simulink model "code_group35"  (R2020a)
settings: Solver=FixedStepAuto  StartTime=0.0  StopTime=10.0  FixedStep=1e-3  RelTol=1e-3  EnableMultiTasking=on
undefined symbols (not defined in the file): A0, A1, D0, D1, D10, D11, D12, D13, D2, D3, D4, D5, D6, D7, D8, D9, PTA0, PTA1, PTA2, PTB2, PTB23, PTB3, PTB9, PTC16, PTC17, PTC2, PTC3, PTC4, PTD0, PTD1, PTD2, PTD3
libraries: frdmk64flib x25, etargetslib x6, dspstat3 x1
settings Model: ExtModeTrigDuration=5  Creator=braed  LastModifiedBy=braed
settings OptimizationCC: EnhancedBackFolding=on  PassReuseOutputArgsAs=Individual arguments  ZeroExternalMemoryAtStartup=off  ZeroInternalMemoryAtStartup=off  MaxStackSize=64  OptimizeBlockOrder=speed  DifferentSizesBufferReuse=on  OptimizationCustomize=off  EfficientTunableParamExpr=on
settings DebuggingCC: ParameterTunabilityLossMsg=error
settings HardwareCC: ProdBitPerPointer=32  ProdBitPerSizeT=32  ProdBitPerPtrDiffT=32  ProdLargestAtomicInteger=Long  ProdLargestAtomicFloat=Double  ProdWordSize=32  ProdHWDeviceType=ARM Compatible->ARM Cortex
settings SFSimCC: MATLABDynamicMemAlloc=off
settings RTWCC: SystemTargetFile=ert.tlc  HardwareBoard=NXP FRDM-K64F  TemplateMakefile=ert_default_tmf  Toolchain=GNU Tools for ARM Embedded Processors
settings CodeAppCC: ForceParamTrailComments=on  IgnoreCustomStorageClasses=off  OperatorAnnotations=on  SimulinkDataObjDesc=on  SFDataObjDesc=on  InsertBlockDesc=on

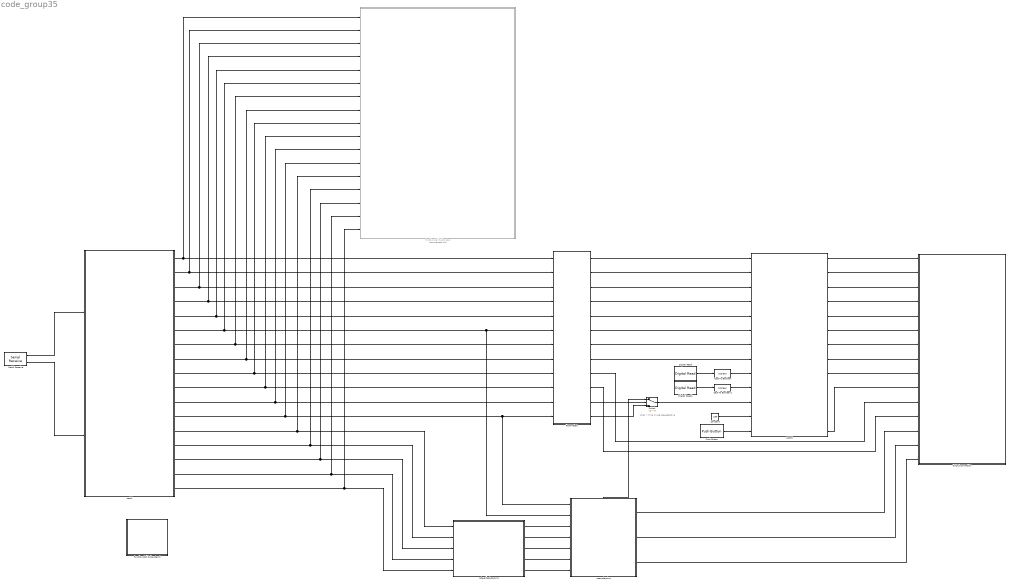
== system code_group35 ==
  note: when > 0 (ie 1) use rate_adaptive
  " Output connection" : Subsystem
  Cast To Boolean : DataTypeConversion  OutDataTypeStr=boolean
  Cast To Boolean1 : DataTypeConversion  OutDataTypeStr=boolean
  Constant : Constant  Value=250
  Digital Read : frdmk64flib/Digital Read  Whichpin=PTC16 (D0)  SampleTime=-1
  Digital Read1 : frdmk64flib/Digital Read  Whichpin=PTC17 (D1)  SampleTime=-1
  Function-Call Subsystem : Subsystem  Commented=on  TreatAsAtomicUnit=on
  Function-Call Subsystem1 : Subsystem  TreatAsAtomicUnit=on
  LOGIC : Stateflow chart  TreatAsAtomicUnit=on
  Parameters : Subsystem
  Push Button : frdmk64flib/Push Button  Whichswitch=SW2  SampleTime1=-1
  Serial Receive : frdmk64flib/Serial Receive  SCIModule=0  Baudrate=uint32(9600)  Parity=None  StopBits=1  HardwareFlowControl=None  ByteOrder=LittleEndian  DataType=uint8  DataLength=28  BlockingMode=off  OutputStatus=on  SampleTime=-1
  Switch : Switch  Criteria=u2 > Threshold
  rate adaptive : Subsystem
      settings: PortSchema="{\"entries\":[{\"content\":{\"sides\":[{\"content\":{\"connectorIds\":[\"In1\",\"In2\",\"In3\",\"In4\",\"In5\",\"In6\",\"In7\"]},\"type\":\"ConnectorPlacement.EquallySpacedRectSide\",\"uuid\":\"63ecb548-1bfe-492b-8fa1-384c5f75ccdd\"},{\"content\":{\"connectorIds\":[\"Out1\",\"Out2\",\"Out3\"],\"side\":\"RIGHT\"},\"type\":\"ConnectorPlacement.EquallySpacedRectSide\",\"uuid\":\"03d354e8-60bf-4739-8c68-3b2530a8d39d\"},{\"content\":{\"connectorIds\":[\"Out4\"],\"side\":\"TOP\"},\"type\":\"ConnectorPlacement.EquallySpacedRectSide\",\"uuid\":\"87bdc17e-9d8d-401e-9bc9-5c1e683b110d\"}]},\"type\":\"ConnectorPlacement.EquallySpacedConnector\",\"uuid\":\"8522751d-691b-4abf-a216-245af807604c\"}],\"packageUris\":[\"http://schema.mathworks.com/mf0/Connector/19700101\"],\"version\":\"1.0\"}"
  rate_adapt_params : Subsystem
  serial : Stateflow chart  TreatAsAtomicUnit=on
  wires:
  LOGIC/7(ATR_GND_CTRL) -> " Output connection"/7(ATR_GND_CTRL)
  Parameters/1(mode_out) -> LOGIC/1(mode)
  Parameters/6(upperInterval) -> LOGIC/6(upper_interval_rate)
  Parameters/7(ARP) -> LOGIC/7(ARP)
  Parameters/8(VRP) -> LOGIC/8(VRP)
  Parameters/5(vent_pulse_amp) -> LOGIC/5(vent_amp)
  Parameters/10(VentSensitivity) -> " Output connection"/12(VENT_CMP_REF_PWM)
  Parameters/2(atr_pulse_width) -> LOGIC/2(atr_pulse_width)
  Parameters/4(vent_pulse_width) -> LOGIC/4(vent_pulse_width)
  Parameters/9(AtrSensitivity) -> " Output connection"/11(ATR_CMP_REF_PWM)
  LOGIC/5(VENT_PACE_CTRL) -> " Output connection"/5(VENT_PACE_CTRL)
  Digital Read/1 -> Cast To Boolean/1
  Digital Read1/1 -> Cast To Boolean1/1
  Parameters/3(atr_pulse_amp) -> LOGIC/3(atr_amp)
  LOGIC/13(FRONTEND_CTRL) -> " Output connection"/10(FRONTEND_CTRL)
  Cast To Boolean/1 -> LOGIC/9(ATR_CMP_DETECT)
  Cast To Boolean1/1 -> LOGIC/10(VENT_CMP_DETECT)
  LOGIC/3(Z_VENT_CTRL) -> " Output connection"/3(Z_VENT_CTRL)
  LOGIC/4(ATR_PACE_CTRL) -> " Output connection"/4(ATR_PACE_CTRL)
  LOGIC/8(VENT_GND_CTRL) -> " Output connection"/8(VENT_GND_CTRL)
  LOGIC/9(PACE_CHARGE_CTRL) -> " Output connection"/9(PACE_CHARGE_CTRL)
  LOGIC/1(PACING_REF_PWM) -> " Output connection"/1(PACING_REF_PWM)
  LOGIC/2(Z_ATR_CTRL) -> " Output connection"/2(Z_ATR_CTRL)
  LOGIC/6(PACE_GND_CTRL) -> " Output connection"/6(PACE_GND_CTRL)
  Serial Receive/1 -> serial/1(rxdata)
  Serial Receive/2 -> serial/2(status)
  rate adaptive/3(led_b) -> " Output connection"/15(B_LED)
  rate adaptive/1(led_r) -> " Output connection"/13(R_LED)
  rate adaptive/2(led_g) -> " Output connection"/14(G_LED)
  Parameters/11(rate_adaptive_out) -> Switch/2
  rate adaptive/4(pacing_rate) -> Switch/1
  Parameters/12(lowerInterval) -> Switch/3
  Switch/1 -> LOGIC/11(lower_interval_rate)
  serial/1(mode) -> Function-Call Subsystem/1(mode), Parameters/1(mode_in)
  serial/2(atr_pw) -> Function-Call Subsystem/2(atr_pw), Parameters/2(atr_pw)
  serial/4(vent_pw) -> Function-Call Subsystem/4(vent_pw), Parameters/4(vent_pw)
  serial/5(vent_amp) -> Function-Call Subsystem/5(vent_amp), Parameters/5(vent_amp)
  serial/6(LRL) -> Function-Call Subsystem/6(LRL), rate adaptive/2(LRL_in), Parameters/6(lowerRateIn)
  serial/7(URL) -> Function-Call Subsystem/7(URL), Parameters/7(upperRateIn)
  serial/8(ARP) -> Function-Call Subsystem/8(ARP), Parameters/8(ARPIn)
  serial/9(VRP) -> Function-Call Subsystem/9(VRP), Parameters/9(VRPIn)
  serial/10(atr_sense) -> Function-Call Subsystem/10(atr_sense), Parameters/10(AtrSensitivityIn)
  serial/11(vent_sense) -> Function-Call Subsystem/11(vent_sense), Parameters/11(VentSensitivityIn)
  serial/12(rate_adp) -> Function-Call Subsystem/12(rate_adp), rate adaptive/1(rate_adaptive_in), Parameters/12(rate_adaptive_in)
  rate_adapt_params/1(MSRout) -> rate adaptive/3(MSR_in)
  rate_adapt_params/2(reac_out) -> rate adaptive/4(reac_time)
  rate_adapt_params/3(recov_out) -> rate adaptive/5(recov_time)
  rate_adapt_params/4(act_thresh_out) -> rate adaptive/6(activity_threshold)
  rate_adapt_params/5(resp_out) -> rate adaptive/7(response_factor)
  serial/13(MSR) -> Function-Call Subsystem/13(MSR), rate_adapt_params/1(MSRin)
  serial/15(recov_t) -> Function-Call Subsystem/15(recov_t), rate_adapt_params/3(recov_in)
  serial/16(act_thresh) -> Function-Call Subsystem/16(act_thresh), rate_adapt_params/4(act_thresh_in)
  serial/17(res_fact) -> Function-Call Subsystem/17(res_fact), rate_adapt_params/5(resp_in)
  serial/3(atr_amp) -> Function-Call Subsystem/3(atr_amp), Parameters/3(atr_amp)
  serial/14(reac_t) -> Function-Call Subsystem/14(reac_t), rate_adapt_params/2(reac_in)
  Constant/1 -> LOGIC/12(AV_Delay)
  Push Button/1 -> LOGIC/13(button)

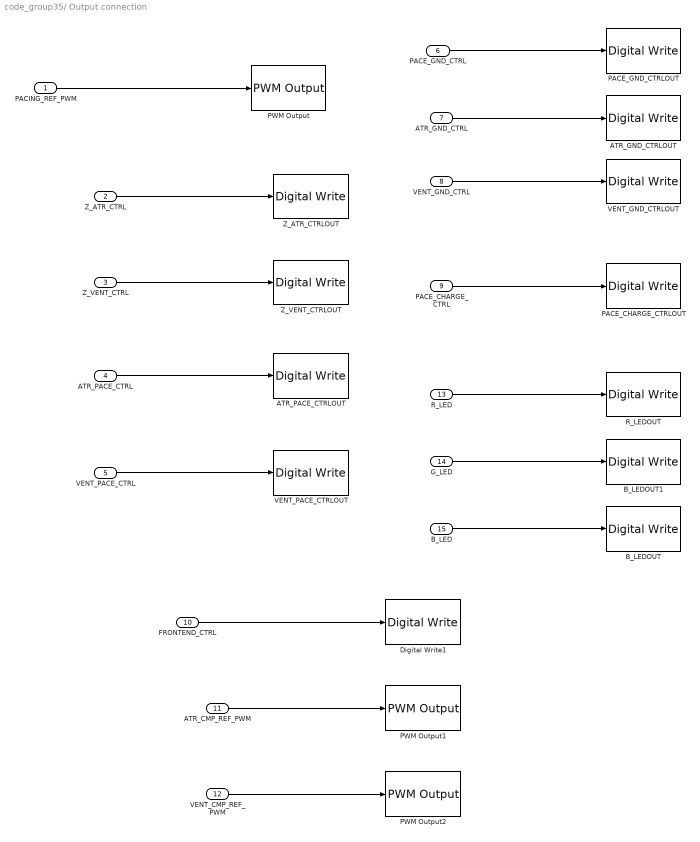
== system code_group35/ Output connection ==
  PACING_REF_PWM : Inport  OutDataTypeStr=uint32
  Z_ATR_CTRL : Inport  Port=2  OutDataTypeStr=uint32
  Z_VENT_CTRL : Inport  Port=3  OutDataTypeStr=uint32
  ATR_PACE_CTRL : Inport  Port=4  OutDataTypeStr=uint32
  VENT_PACE_CTRL : Inport  Port=5  OutDataTypeStr=uint32
  PACE_GND_CTRL : Inport  Port=6  OutDataTypeStr=uint32
  ATR_GND_CTRL : Inport  Port=7  OutDataTypeStr=uint32
  VENT_GND_CTRL : Inport  Port=8  OutDataTypeStr=uint32
  PACE_CHARGE_CTRL : Inport  Port=9  OutDataTypeStr=uint32
  FRONTEND_CTRL : Inport  Port=10  OutDataTypeStr=uint8
  ATR_CMP_REF_PWM : Inport  Port=11  OutDataTypeStr=uint32
  VENT_CMP_REF_PWM : Inport  Port=12  OutDataTypeStr=uint32
  R_LED : Inport  Port=13  OutDataTypeStr=uint32
  G_LED : Inport  Port=14  OutDataTypeStr=uint32
  B_LED : Inport  Port=15  OutDataTypeStr=uint32
  ATR_GND_CTRLOUT : frdmk64flib/Digital Write  Whichpin=PTD2 (D11)
  ATR_PACE_CTRLOUT : frdmk64flib/Digital Write  Whichpin=PTA0 (D8)
  B_LEDOUT : frdmk64flib/Digital Write  Whichpin=BLUE_LED
  B_LEDOUT1 : frdmk64flib/Digital Write  Whichpin=GREEN_LED
  Digital Write1 : frdmk64flib/Digital Write  Whichpin=PTD1 (D13)
  PACE_CHARGE_CTRLOUT : frdmk64flib/Digital Write  Whichpin=PTB9 (D2)
  PACE_GND_CTRLOUT : frdmk64flib/Digital Write  Whichpin=PTD0 (D10)
  PWM Output : frdmk64flib/PWM Output  Whichpin=PTA2 (D5)  InitialFrequency=2000  InitialDutyCycle=30
  PWM Output1 : frdmk64flib/PWM Output  Whichpin=PTC2 (D6)  InitialFrequency=2000  InitialDutyCycle=30
  PWM Output2 : frdmk64flib/PWM Output  Whichpin=PTA1 (D3)  InitialFrequency=2000  InitialDutyCycle=30
  R_LEDOUT : frdmk64flib/Digital Write  Whichpin=RED_LED
  VENT_GND_CTRLOUT : frdmk64flib/Digital Write  Whichpin=PTD3 (D12)
  VENT_PACE_CTRLOUT : frdmk64flib/Digital Write  Whichpin=PTC4 (D9)
  Z_ATR_CTRLOUT : frdmk64flib/Digital Write  Whichpin=PTB23 (D4)
  Z_VENT_CTRLOUT : frdmk64flib/Digital Write  Whichpin=PTC3 (D7)
  wires:
  PACING_REF_PWM/1 -> PWM Output/1
  Z_VENT_CTRL/1 -> Z_VENT_CTRLOUT/1
  PACE_GND_CTRL/1 -> PACE_GND_CTRLOUT/1
  Z_ATR_CTRL/1 -> Z_ATR_CTRLOUT/1
  ATR_PACE_CTRL/1 -> ATR_PACE_CTRLOUT/1
  VENT_GND_CTRL/1 -> VENT_GND_CTRLOUT/1
  B_LED/1 -> B_LEDOUT/1
  PACE_CHARGE_CTRL/1 -> PACE_CHARGE_CTRLOUT/1
  ATR_GND_CTRL/1 -> ATR_GND_CTRLOUT/1
  G_LED/1 -> B_LEDOUT1/1
  R_LED/1 -> R_LEDOUT/1
  VENT_PACE_CTRL/1 -> VENT_PACE_CTRLOUT/1
  VENT_CMP_REF_PWM/1 -> PWM Output2/1
  ATR_CMP_REF_PWM/1 -> PWM Output1/1
  FRONTEND_CTRL/1 -> Digital Write1/1

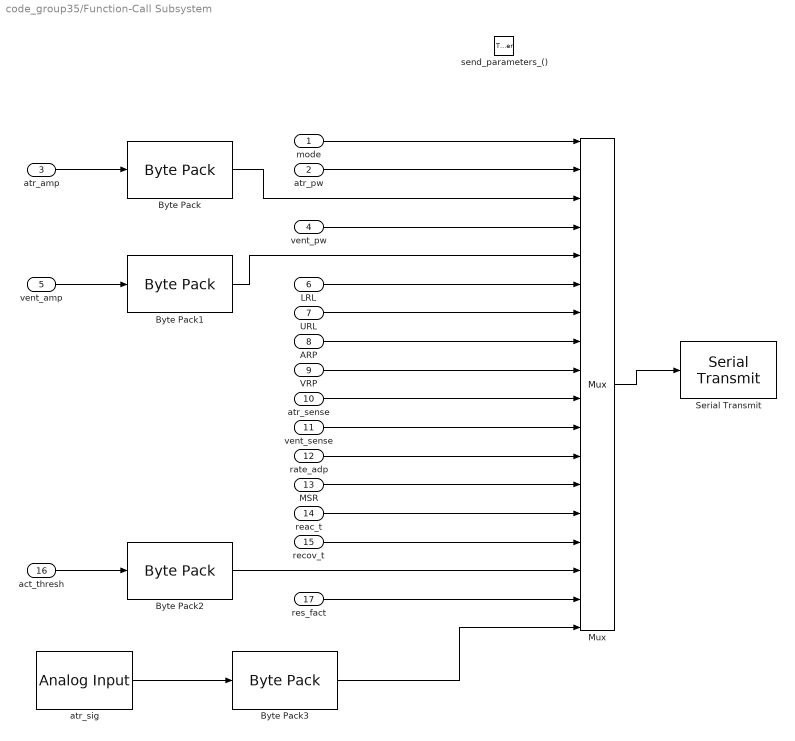
== system code_group35/Function-Call Subsystem ==
  mode : Inport
  atr_pw : Inport  Port=2
  atr_amp : Inport  Port=3
  vent_pw : Inport  Port=4
  vent_amp : Inport  Port=5
  LRL : Inport  Port=6
  URL : Inport  Port=7
  ARP : Inport  Port=8
  VRP : Inport  Port=9
  atr_sense : Inport  Port=10
  vent_sense : Inport  Port=11
  rate_adp : Inport  Port=12
  MSR : Inport  Port=13
  reac_t : Inport  Port=14
  recov_t : Inport  Port=15
  act_thresh : Inport  Port=16
  res_fact : Inport  Port=17
  send_parameters_() : TriggerPort  TriggerType=function-call  IsSimulinkFunction=on  FunctionName=send_parameters_  VariantControl=Variant
  Byte Pack : etargetslib/Byte Pack  datatypes={'single'}  byteAlign=1
  Byte Pack1 : etargetslib/Byte Pack  datatypes={'single'}  byteAlign=1
  Byte Pack2 : etargetslib/Byte Pack  datatypes={'single'}  byteAlign=1
  Byte Pack3 : etargetslib/Byte Pack  datatypes={'double'}  byteAlign=1
  Mux : Mux  Inputs=18
  Serial Transmit : frdmk64flib/Serial Transmit  SCIModule=0  Baudrate=uint32(9600)  Parity=None  StopBits=1  HardwareFlowControl=None  ByteOrder=LittleEndian  BlockingMode=on  OutputStatus=off
  atr_sig : frdmk64flib/Analog Input  Whichpin=PTB2 (A0)  SampleTime=-1
  wires:
  mode/1 -> Mux/1
  Mux/1 -> Serial Transmit/1
  atr_pw/1 -> Mux/2
  atr_amp/1 -> Byte Pack/1
  Byte Pack/1 -> Mux/3
  vent_pw/1 -> Mux/4
  LRL/1 -> Mux/6
  URL/1 -> Mux/7
  ARP/1 -> Mux/8
  VRP/1 -> Mux/9
  atr_sense/1 -> Mux/10
  vent_sense/1 -> Mux/11
  rate_adp/1 -> Mux/12
  MSR/1 -> Mux/13
  reac_t/1 -> Mux/14
  recov_t/1 -> Mux/15
  act_thresh/1 -> Byte Pack2/1
  res_fact/1 -> Mux/17
  Byte Pack1/1 -> Mux/5
  vent_amp/1 -> Byte Pack1/1
  Byte Pack2/1 -> Mux/16
  atr_sig/1 -> Byte Pack3/1
  Byte Pack3/1 -> Mux/18

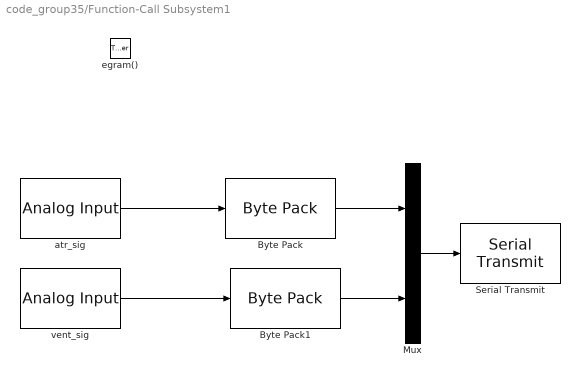
== system code_group35/Function-Call Subsystem1 ==
  egram() : TriggerPort  TriggerType=function-call  IsSimulinkFunction=on  FunctionName=egram_double  VariantControl=Variant
  Byte Pack : etargetslib/Byte Pack  datatypes={'double'}  byteAlign=1
  Byte Pack1 : etargetslib/Byte Pack  datatypes={'double'}  byteAlign=1
  Mux : Mux  Inputs=2
  Serial Transmit : frdmk64flib/Serial Transmit  SCIModule=0  Baudrate=uint32(9600)  Parity=None  StopBits=1  HardwareFlowControl=None  ByteOrder=LittleEndian  BlockingMode=on  OutputStatus=off
  atr_sig : frdmk64flib/Analog Input  Whichpin=PTB2 (A0)  SampleTime=-1
  vent_sig : frdmk64flib/Analog Input  Whichpin=PTB3 (A1)  SampleTime=-1
  wires:
  Mux/1 -> Serial Transmit/1
  atr_sig/1 -> Byte Pack/1
  vent_sig/1 -> Byte Pack1/1
  Byte Pack1/1 -> Mux/2
  Byte Pack/1 -> Mux/1

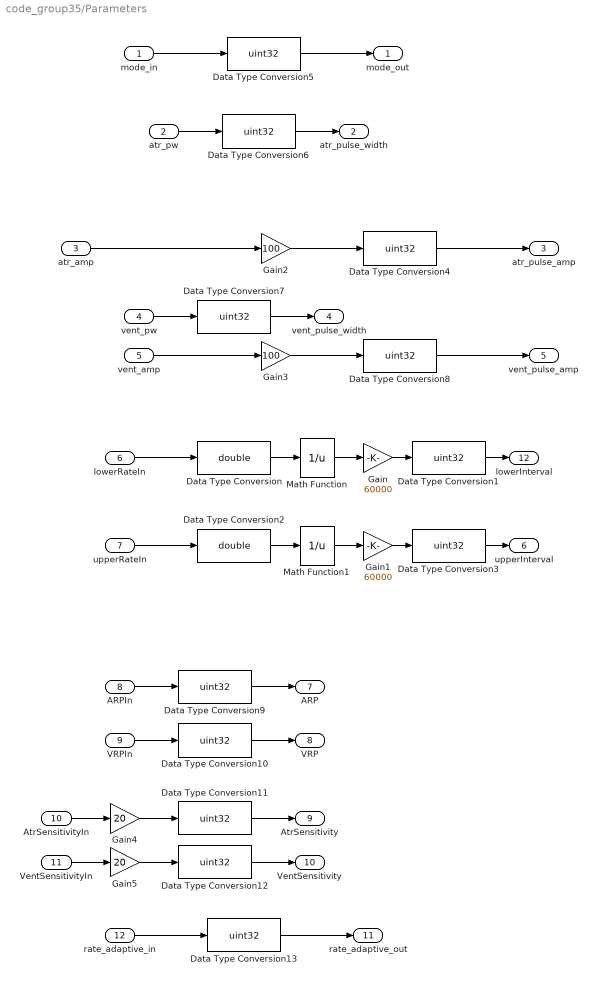
== system code_group35/Parameters ==
  mode_in : Inport  OutDataTypeStr=uint8
  atr_pw : Inport  Port=2  OutDataTypeStr=uint8
  atr_amp : Inport  Port=3  OutDataTypeStr=single
  vent_pw : Inport  Port=4  OutDataTypeStr=uint8
  vent_amp : Inport  Port=5  OutDataTypeStr=single
  lowerRateIn : Inport  Port=6  OutDataTypeStr=uint8  Unit=ppm
  upperRateIn : Inport  Port=7  OutDataTypeStr=uint8  Unit=ppm
  ARPIn : Inport  Port=8  OutDataTypeStr=uint8
  VRPIn : Inport  Port=9  OutDataTypeStr=uint8
  AtrSensitivityIn : Inport  Port=10  OutDataTypeStr=uint8
  VentSensitivityIn : Inport  Port=11  OutDataTypeStr=uint8
  rate_adaptive_in : Inport  Port=12  OutDataTypeStr=uint8
  Data Type Conversion : DataTypeConversion  OutDataTypeStr=double
  Data Type Conversion1 : DataTypeConversion  OutDataTypeStr=uint32
  Data Type Conversion{4..13} (10 alike) : DataTypeConversion  OutDataTypeStr=uint32  RndMeth=Round
  Data Type Conversion2 : DataTypeConversion  OutDataTypeStr=double
  Data Type Conversion3 : DataTypeConversion  OutDataTypeStr=uint32
  Gain : Gain  Gain=60000  OutDataTypeStr=double
  Gain1 : Gain  Gain=60000  OutDataTypeStr=double
  Gain2 : Gain  Gain=100  OutDataTypeStr=single
  Gain3 : Gain  Gain=100
  Gain4 : Gain  Gain=20
  Gain5 : Gain  Gain=20
  Math Function : Math  Operator=reciprocal  SaturateOnIntegerOverflow=on
  Math Function1 : Math  Operator=reciprocal  SaturateOnIntegerOverflow=on
  mode_out : Outport  OutDataTypeStr=uint32  Unit=ms
  atr_pulse_width : Outport  Port=2  OutDataTypeStr=uint32  Unit=ms
  atr_pulse_amp : Outport  Port=3  OutDataTypeStr=uint32  Unit=mV
  vent_pulse_width : Outport  Port=4  OutDataTypeStr=uint32  Unit=ms
  vent_pulse_amp : Outport  Port=5  OutDataTypeStr=uint32  Unit=mV
  upperInterval : Outport  Port=6  OutDataTypeStr=uint32  Unit=ms
  ARP : Outport  Port=7  OutDataTypeStr=uint32
  VRP : Outport  Port=8  OutDataTypeStr=uint32
  AtrSensitivity : Outport  Port=9  OutDataTypeStr=uint32
  VentSensitivity : Outport  Port=10  OutDataTypeStr=uint32
  rate_adaptive_out : Outport  Port=11  OutDataTypeStr=uint32  Unit=ms
  lowerInterval : Outport  Port=12  OutDataTypeStr=uint32  Unit=ms
  wires:
  Math Function/1 -> Gain/1
  Gain/1 -> Data Type Conversion1/1
  lowerRateIn/1 -> Data Type Conversion/1
  Math Function1/1 -> Gain1/1
  upperRateIn/1 -> Data Type Conversion2/1
  Gain1/1 -> Data Type Conversion3/1
  VRPIn/1 -> Data Type Conversion10/1
  ARPIn/1 -> Data Type Conversion9/1
  Data Type Conversion/1 -> Math Function/1
  Data Type Conversion1/1 -> lowerInterval/1
  Data Type Conversion2/1 -> Math Function1/1
  Data Type Conversion3/1 -> upperInterval/1
  Gain2/1 -> Data Type Conversion4/1
  Data Type Conversion4/1 -> atr_pulse_amp/1
  Data Type Conversion8/1 -> vent_pulse_amp/1
  Gain3/1 -> Data Type Conversion8/1
  vent_amp/1 -> Gain3/1
  rate_adaptive_in/1 -> Data Type Conversion13/1
  atr_amp/1 -> Gain2/1
  mode_in/1 -> Data Type Conversion5/1
  Data Type Conversion5/1 -> mode_out/1
  atr_pw/1 -> Data Type Conversion6/1
  Data Type Conversion6/1 -> atr_pulse_width/1
  vent_pw/1 -> Data Type Conversion7/1
  Data Type Conversion7/1 -> vent_pulse_width/1
  Data Type Conversion9/1 -> ARP/1
  Data Type Conversion10/1 -> VRP/1
  Data Type Conversion11/1 -> AtrSensitivity/1
  Data Type Conversion12/1 -> VentSensitivity/1
  Data Type Conversion13/1 -> rate_adaptive_out/1
  VentSensitivityIn/1 -> Gain5/1
  AtrSensitivityIn/1 -> Gain4/1
  Gain4/1 -> Data Type Conversion11/1
  Gain5/1 -> Data Type Conversion12/1

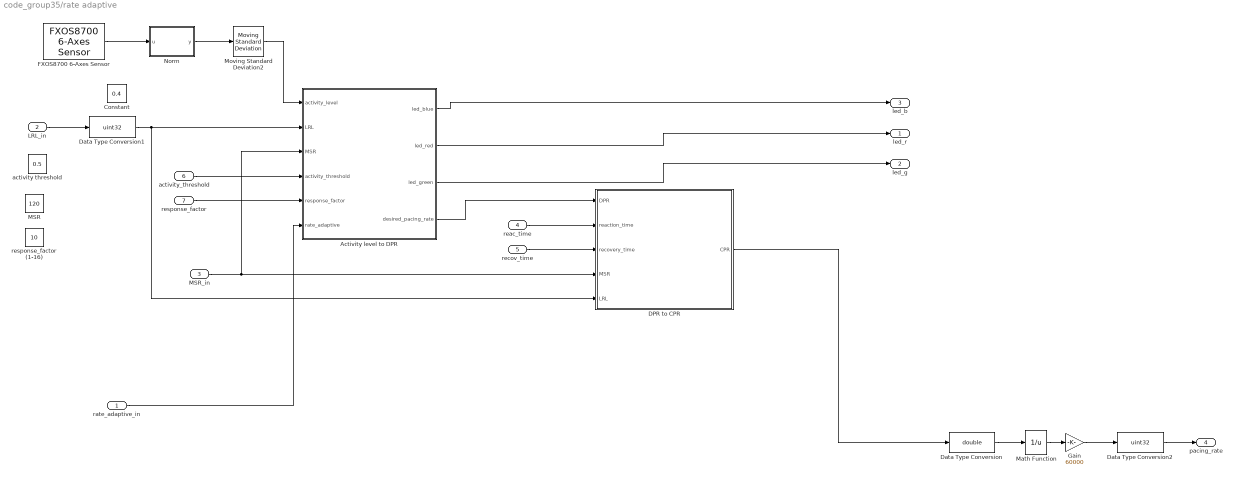
== system code_group35/rate adaptive ==
  rate_adaptive_in : Inport  OutDataTypeStr=uint8
  LRL_in : Inport  Port=2  OutDataTypeStr=uint8
  MSR_in : Inport  Port=3  OutDataTypeStr=uint32
  reac_time : Inport  Port=4  OutDataTypeStr=uint32
  recov_time : Inport  Port=5  OutDataTypeStr=uint32
  activity_threshold : Inport  Port=6  OutDataTypeStr=double
  response_factor : Inport  Port=7  OutDataTypeStr=uint32
  Activity level to DPR : Stateflow chart  TreatAsAtomicUnit=on
      settings: PortSchema="{\"entries\":[{\"content\":{\"sides\":[{\"content\":{\"connectorIds\":[\"In1\",\"In2\",\"In4\",\"In3\",\"In5\",\"In6\"]},\"type\":\"ConnectorPlacement.EquallySpacedRectSide\",\"uuid\":\"64c79778-1dae-454c-adeb-b2b27c3ff420\"},{\"content\":{\"connectorIds\":[\"Out1\",\"Out2\",\"Out3\",\"Out4\"],\"side\":\"RIGHT\"},\"type\":\"ConnectorPlacement.EquallySpacedRectSide\",\"uuid\":\"c97016c6-8fdd-40e3-ba17-a509eff469e8\"},{\"content\":{\"connectorIds\":[],\"side\":\"TOP\"},\"type\":\"ConnectorPlacement.EquallySpacedRectSide\",\"uuid\":\"7272e5a5-3a89-40ce-82da-b41993aad90e\"}]},\"type\":\"ConnectorPlacement.EquallySpacedConnector\",\"uuid\":\"8a580f9c-8073-46c4-ba85-130e20a78434\"}],\"packageUris\":[\"http://schema.mathworks.com/mf0/Connector/19700101\"],\"version\":\"1.0\"}"
  Constant : Constant  Value=0.4
  DPR to CPR : Stateflow chart  TreatAsAtomicUnit=on
  Data Type Conversion : DataTypeConversion  OutDataTypeStr=double
  Data Type Conversion1 : DataTypeConversion  OutDataTypeStr=uint32
  Data Type Conversion2 : DataTypeConversion  OutDataTypeStr=uint32
  FXOS8700 6-Axes Sensor : frdmk64flib/FXOS8700 6-Axes Sensor  Activesensor=Accelerometer only  ODR=100Hz  HybridODR=400Hz  Accelfullrange=-4g to +4g  SampleTime=1/100
  Gain : Gain  Gain=60000  OutDataTypeStr=double
  MSR : Constant  Value=120  OutDataTypeStr=uint32
  Math Function : Math  Operator=reciprocal  SaturateOnIntegerOverflow=on
  Moving Standard Deviation2 : dspstat3/Moving Standard Deviation  Method=Sliding window  ForgettingFactorPort=off  SpecifyWindowLength=on  WindowLength=100  ForgettingFactor=0.9  SimulateUsing=Code generation
      settings: SourceProductBaseCode=DS
  Norm : MATLAB Function  TreatAsAtomicUnit=on
  activity threshold : Constant  Value=0.5  OutDataTypeStr=double
  response_factor (1-16) : Constant  Value=10  OutDataTypeStr=uint32
  led_r : Outport  OutDataTypeStr=uint32  Unit=ms
  led_g : Outport  Port=2  OutDataTypeStr=uint32  Unit=ms
  led_b : Outport  Port=3  OutDataTypeStr=uint32  Unit=ms
  pacing_rate : Outport  Port=4  OutDataTypeStr=uint32  Unit=ms
  wires:
  Norm/1(y) -> Moving Standard Deviation2/1
  Activity level to DPR/1(led_blue) -> led_b/1
  FXOS8700 6-Axes Sensor/1 -> Norm/1(u)
  rate_adaptive_in/1 -> Activity level to DPR/6(rate_adaptive)
  LRL_in/1 -> Data Type Conversion1/1
  Math Function/1 -> Gain/1
  Activity level to DPR/4(desired_pacing_rate) -> DPR to CPR/1(DPR)
  MSR_in/1 -> Activity level to DPR/4(MSR), DPR to CPR/4(MSR)
  reac_time/1 -> DPR to CPR/2(reaction_time)
  recov_time/1 -> DPR to CPR/3(recovery_time)
  Activity level to DPR/2(led_red) -> led_r/1
  Activity level to DPR/3(led_green) -> led_g/1
  response_factor/1 -> Activity level to DPR/5(response_factor)
  Gain/1 -> Data Type Conversion2/1
  Data Type Conversion2/1 -> pacing_rate/1
  activity_threshold/1 -> Activity level to DPR/3(activity_threshold)
  Moving Standard Deviation2/1 -> Activity level to DPR/1(activity_level)
  DPR to CPR/1(CPR) -> Data Type Conversion/1
  Data Type Conversion/1 -> Math Function/1
  Data Type Conversion1/1 -> DPR to CPR/5(LRL), Activity level to DPR/2(LRL)

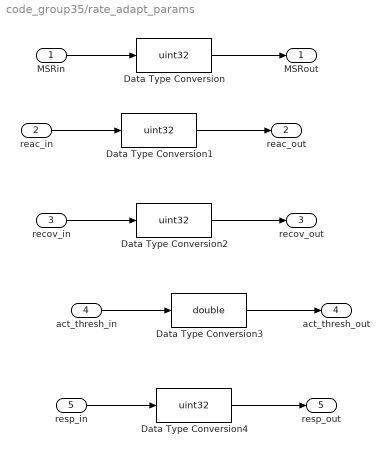
== system code_group35/rate_adapt_params ==
  MSRin : Inport  OutDataTypeStr=uint8
  reac_in : Inport  Port=2  OutDataTypeStr=uint8
  recov_in : Inport  Port=3  OutDataTypeStr=uint8
  act_thresh_in : Inport  Port=4  OutDataTypeStr=single
  resp_in : Inport  Port=5  OutDataTypeStr=uint8
  Data Type Conversion{,1..2,4} (4 alike) : DataTypeConversion  OutDataTypeStr=uint32
  Data Type Conversion3 : DataTypeConversion  OutDataTypeStr=double
  MSRout : Outport  OutDataTypeStr=uint32
  reac_out : Outport  Port=2  OutDataTypeStr=uint32
  recov_out : Outport  Port=3  OutDataTypeStr=uint32
  act_thresh_out : Outport  Port=4  OutDataTypeStr=double
  resp_out : Outport  Port=5  OutDataTypeStr=uint32
  wires:
  MSRin/1 -> Data Type Conversion/1
  Data Type Conversion/1 -> MSRout/1
  Data Type Conversion1/1 -> reac_out/1
  reac_in/1 -> Data Type Conversion1/1
  Data Type Conversion2/1 -> recov_out/1
  recov_in/1 -> Data Type Conversion2/1
  Data Type Conversion3/1 -> act_thresh_out/1
  act_thresh_in/1 -> Data Type Conversion3/1
  Data Type Conversion4/1 -> resp_out/1
  resp_in/1 -> Data Type Conversion4/1

== stateflow chart code_group35/serial ==
  settings: executeAtInitialization=1
  state SET_PARAMS
    entry:
    mode = cast(rxdata(3),'uint8');
    atr_pw = cast(rxdata(4),'uint8');
    atr_amp = typecast(rxdata(5:8),'single'); %single
    vent_pw = cast(rxdata(9),'uint8');
    vent_amp = typecast(rxdata(10:13),'single'); %single
    LRL = cast(rxdata(14),'uint8');
    URL = cast(rxdata(15),'uint8');
    ARP = cast(rxdata(16),'uint8');
    VRP = cast(rxdata(17),'uint8');
    atr_sense = cast(rxdata(18),'uint8');
    vent_sense = cast(rxdata(19),'uint8');
    rate_adp = cast(rxdata(20),'uint8');
    MSR = cast(rxdata(21),'uint8');
    reac_t = cast(rxdata(22),'uint8');
    recov_t = cast(rxdata(23),'uint8');
    act_thresh = typecast(rxdata(24:27),'single'); %single
    res_fact = cast(rxdata(28),'uint8');
  state INITIAL
    entry:
    mode = 0;
    atr_pw = 20;
    atr_amp = cast(1,'single');
    vent_pw = 20;
    vent_amp = cast(1,'single');
    LRL = 60;
    URL = 60;
    ARP = 20;
    VRP = 20;
    atr_sense = 4;
    vent_sense = 4;
    rate_adp = 1;
    MSR = 120;
    reac_t = 30;
    recov_t = 30;
    act_thresh = cast(0.5,'single');
    res_fact = 10;
  state STANDBY
    %wait
  state EGRAM_MODE
    entry:
    egram_double();
  state ECHO_PARAM
    entry:
    %send_parameters_();
  SET_PARAMS -> STANDBY
  (default) -> INITIAL
  (junction 10) -> STANDBY [order 2]
  (junction 12) -> SET_PARAMS [order 1] : [rxdata(2) == hex2dec('13')]
  INITIAL -> STANDBY
  STANDBY -> (junction 10) : [status == 0]
  (junction 10) -> (junction 12) [order 1] : [rxdata(1) == hex2dec('16')]
  (junction 12) -> EGRAM_MODE [order 3] : [rxdata(2) == hex2dec('47')]
  (junction 12) -> ECHO_PARAM [order 2] : [rxdata(2) == hex2dec('22')]
  ECHO_PARAM -> STANDBY
  EGRAM_MODE -> STANDBY
  data: mode output uint8; atr_pw output uint8; atr_amp output single; vent_pw output uint8; vent_amp output single; LRL output uint8; URL output uint8; rxdata input uint8; status input uint8; ARP output uint8; VRP output uint8; atr_sense output uint8; vent_sense output uint8; rate_adp output uint8; MSR output uint8; reac_t output uint8; recov_t output uint8; act_thresh output single; res_fact output uint8

== stateflow chart code_group35/rate adaptive/Activity level to DPR ==
  state Sprinting
    led_blue = 0
    led_green = 0
    led_red = 1
    desired_pacing_rate = LRL + (2*response_factor)
    if( desired_pacing_rate > MSR)
    desired_pacing_rate = MSR
    end
  state START
    %check if rate_adaptive is on
  state walking
    led_blue = 0
    led_green = 1
    led_red = 0
    desired_pacing_rate = LRL
  state Running
    led_blue = 1
    led_green = 0
    led_red = 0
    desired_pacing_rate = LRL + response_factor
    if( desired_pacing_rate > MSR)
    desired_pacing_rate = MSR
    end
  walking -> Sprinting [order 2] : [activity_level > (2*activity_threshold)]
  (default) -> START
  START -> walking : [rate_adaptive == 1]
  Sprinting -> walking [order 1] : [activity_level < activity_threshold]
  Running -> walking [order 2] : [activity_level < activity_threshold]
  Sprinting -> Running [order 2] : [activity_level < (2*activity_threshold)]
  Running -> Sprinting [order 1] : [activity_level > (2*activity_threshold)]
  walking -> Running [order 1] : [activity_level > activity_threshold]
  data: activity_level input; led_blue output; led_red output; led_green output; desired_pacing_rate output uint32; LRL input; activity_threshold input; MSR input; response_factor input; rate_adaptive input

== stateflow chart code_group35/LOGIC ==
  state DDD
    note: Dont pulse if detected
    note: Dont pulse if detected
    state Charging [commented out]
      PACE_CHARGE_CTRL = 1;
      PACE_GND_CTRL = 1;
      Z_ATR_CTRL = 0;
      Z_VENT_CTRL = 0;
      PACING_REF_PWM = (atr_amp);
      VENT_PACE_CTRL = 0;
      ATR_PACE_CTRL = 0;
      VENT_GND_CTRL = 0;
      ATR_GND_CTRL = 1;
    state Charging1 [commented out]
      PACE_CHARGE_CTRL = 1;
      PACE_GND_CTRL = 1;
      Z_ATR_CTRL = 0;
      Z_VENT_CTRL = 0;
      PACING_REF_PWM = (vent_amp);
      VENT_PACE_CTRL = 0;
      ATR_PACE_CTRL = 0;
      ATR_GND_CTRL = 0;
      VENT_GND_CTRL = 1;
    state Discharging1 [commented out]
      PACE_CHARGE_CTRL = 0;
      PACE_GND_CTRL = 1;
      VENT_GND_CTRL = 0;
      ATR_GND_CTRL = 0;
      ATR_PACE_CTRL = 0;
      VENT_PACE_CTRL = 1;
    state Charging3
      PACE_CHARGE_CTRL = 1;
      PACE_GND_CTRL = 1;
      Z_ATR_CTRL = 0;
      Z_VENT_CTRL = 0;
      PACING_REF_PWM = (vent_amp);
      VENT_PACE_CTRL = 0;
      ATR_PACE_CTRL = 0;
      ATR_GND_CTRL = 0;
      VENT_GND_CTRL = 1;
    state Charging2
      PACE_CHARGE_CTRL = 1;
      PACE_GND_CTRL = 1;
      Z_ATR_CTRL = 0;
      Z_VENT_CTRL = 0;
      PACING_REF_PWM = (atr_amp);
      VENT_PACE_CTRL = 0;
      ATR_PACE_CTRL = 0;
      VENT_GND_CTRL = 0;
      ATR_GND_CTRL = 1;
    state Discharging
      PACE_CHARGE_CTRL = 0;
      PACE_GND_CTRL = 1;
      VENT_GND_CTRL = 0;
      ATR_GND_CTRL = 0;
      VENT_PACE_CTRL = 0;
      ATR_PACE_CTRL = 1;
    state Discharging2
      PACE_CHARGE_CTRL = 0;
      PACE_GND_CTRL = 1;
      VENT_GND_CTRL = 0;
      ATR_GND_CTRL = 0;
      ATR_PACE_CTRL = 0;
      VENT_PACE_CTRL = 1;
    (junction 324) -> DDD.Charging [commented out] : [ATR_CMP_DETECT == 1]
    (junction 325) -> Charging1 [commented out] : [VENT_CMP_DETECT == 1]
    DDD.Charging -> (junction 324) [commented out] : after(ARP - atr_pulse_width, msec)
    (junction 324) -> ? [commented out] : after(lower_interval_rate-ARP,msec)[ATR_CMP_DETECT == 0]
    Charging1 -> (junction 325) [commented out] : after(VRP - vent_pulse_width, msec)
    (junction 325) -> Discharging1 [commented out] : after(lower_interval_rate-VRP,msec)[VENT_CMP_DETECT == 0]
    (default) -> DDD.Charging [commented out] : [after(atr_pulse_width, msec)]
    Discharging1 -> Charging1 [commented out] : [after(vent_pulse_width, msec)]
    DDD.Charging2 -> (junction 354) [order 1] : [button == true]
    (junction 354) -> DDD.Discharging : [after(lower_interval_rate-ARP,msec)]
    DDD.Charging3 -> DDD.Discharging2 [order 2] : [VENT_CMP_DETECT == 1]
    DDD.Charging2 -> DDD.Discharging [order 3]
    (default) -> DDD.Discharging
    DDD.Discharging2 -> DDD.Charging3 : [after(vent_pulse_width,msec)]
    DDD.Discharging -> DDD.Charging2 : [after(atr_pulse_width,msec)]
    DDD.Charging2 -> DDD.Discharging2 [order 2] : [button == false && after(AV_Delay,msec)]
    DDD.Charging3 -> DDD.Discharging [order 1] : [after((lower_interval_rate-atr_pulse_width)-AV_Delay-vent_pulse_width,msec)]
    DDD.Charging3 -> DDD.Charging2 [order 3] : [ATR_CMP_DETECT == 1]
  state AAI
    note: Dont pulse if detected
    state Charging
      PACE_CHARGE_CTRL = 1;
      PACE_GND_CTRL = 1;
      Z_ATR_CTRL = 0;
      Z_VENT_CTRL = 0;
      PACING_REF_PWM = (atr_amp);
      VENT_PACE_CTRL = 0;
      ATR_PACE_CTRL = 0;
      VENT_GND_CTRL = 0;
      ATR_GND_CTRL = 1;
    state Discharging
      PACE_CHARGE_CTRL = 0;
      PACE_GND_CTRL = 1;
      VENT_GND_CTRL = 0;
      ATR_GND_CTRL = 0;
      VENT_PACE_CTRL = 0;
      ATR_PACE_CTRL = 1;
    (junction 195) -> AAI.Charging [order 1] : [ATR_CMP_DETECT == 1]
    (default) -> AAI.Charging
    AAI.Charging -> (junction 195) : after(ARP - atr_pulse_width, msec)
    (junction 195) -> AAI.Discharging [order 2] : after(lower_interval_rate-ARP,msec)[ATR_CMP_DETECT == 0]
    AAI.Discharging -> AAI.Charging : [after(atr_pulse_width, msec)]
  state VVI
    note: Dont pulse if detected
    state Charging
      PACE_CHARGE_CTRL = 1;
      PACE_GND_CTRL = 1;
      Z_ATR_CTRL = 0;
      Z_VENT_CTRL = 0;
      PACING_REF_PWM = (vent_amp);
      VENT_PACE_CTRL = 0;
      ATR_PACE_CTRL = 0;
      ATR_GND_CTRL = 0;
      VENT_GND_CTRL = 1;
    state Discharging
      PACE_CHARGE_CTRL = 0;
      PACE_GND_CTRL = 1;
      VENT_GND_CTRL = 0;
      ATR_GND_CTRL = 0;
      ATR_PACE_CTRL = 0;
      VENT_PACE_CTRL = 1;
    (junction 179) -> VVI.Charging [order 1] : [VENT_CMP_DETECT == 1]
    (default) -> VVI.Charging
    VVI.Charging -> (junction 179) : after(VRP - vent_pulse_width, msec)
    (junction 179) -> VVI.Discharging [order 2] : after(lower_interval_rate-VRP,msec)[VENT_CMP_DETECT == 0]
    VVI.Discharging -> VVI.Charging : [after(vent_pulse_width, msec)]
  note: Initial state to set parameters and grounds for safety
  state INIT
    if(mode == 1 | mode == 3)
    PACING_REF_PWM = (atr_amp);
    LED_STATE_RED = 1;
    LED_STATE_GREEN = 0;
    LED_STATE_BLUE = 0;
    else
    PACING_REF_PWM = (vent_amp);
    LED_STATE_RED = 0;
    LED_STATE_GREEN = 1;
    LED_STATE_BLUE = 0;
    end
    Z_ATR_CTRL = 0;
    Z_VENT_CTRL = 0;
    ATR_PACE_CTRL = 0;
    VENT_PACE_CTRL = 0;
    PACE_GND_CTRL = 1;
    ATR_GND_CTRL = 0;
    VENT_GND_CTRL = 0;
    PACE_CHARGE_CTRL = 1;
    FRONTEND_CTRL = 1;
  state AOO
    state Charging
      PACE_CHARGE_CTRL = 1;
      PACE_GND_CTRL = 1;
      Z_ATR_CTRL = 0;
      Z_VENT_CTRL = 0;
      PACING_REF_PWM = (atr_amp);
      ATR_PACE_CTRL = 0;
      VENT_PACE_CTRL = 0;
      VENT_GND_CTRL = 0;
      ATR_GND_CTRL = 1;
    state Discharging
      PACE_CHARGE_CTRL = 0;
      PACE_GND_CTRL = 1;
      ATR_GND_CTRL = 0;
      VENT_GND_CTRL = 0;
      VENT_PACE_CTRL = 0;
      ATR_PACE_CTRL = 1;
    (default) -> AOO.Charging
    AOO.Charging -> AOO.Discharging : [after(lower_interval_rate - atr_pulse_width, msec)]
    AOO.Discharging -> AOO.Charging : [after(atr_pulse_width, msec)]
  state VOO
    state Charging
      PACE_CHARGE_CTRL = 1;
      PACE_GND_CTRL = 1;
      Z_ATR_CTRL = 0;
      Z_VENT_CTRL = 0;
      PACING_REF_PWM = (vent_amp);
      VENT_PACE_CTRL = 0;
      ATR_PACE_CTRL = 0;
      ATR_GND_CTRL = 0;
      VENT_GND_CTRL = 1;
    state Discharging
      PACE_CHARGE_CTRL = 0;
      PACE_GND_CTRL = 1;
      VENT_GND_CTRL = 0;
      ATR_GND_CTRL = 0;
      ATR_PACE_CTRL = 0;
      VENT_PACE_CTRL = 1;
    (default) -> VOO.Charging
    VOO.Charging -> VOO.Discharging : [after(lower_interval_rate - vent_pulse_width, msec)]
    VOO.Discharging -> VOO.Charging : [after(vent_pulse_width, msec)]
  state DOO
    state Charging3
      PACE_CHARGE_CTRL = 1;
      PACE_GND_CTRL = 1;
      Z_ATR_CTRL = 0;
      Z_VENT_CTRL = 0;
      PACING_REF_PWM = (vent_amp);
      VENT_PACE_CTRL = 0;
      ATR_PACE_CTRL = 0;
      ATR_GND_CTRL = 0;
      VENT_GND_CTRL = 1;
    state Charging2
      PACE_CHARGE_CTRL = 1;
      PACE_GND_CTRL = 1;
      Z_ATR_CTRL = 0;
      Z_VENT_CTRL = 0;
      PACING_REF_PWM = (atr_amp);
      VENT_PACE_CTRL = 0;
      ATR_PACE_CTRL = 0;
      VENT_GND_CTRL = 0;
      ATR_GND_CTRL = 1;
    state Discharging
      PACE_CHARGE_CTRL = 0;
      PACE_GND_CTRL = 1;
      VENT_GND_CTRL = 0;
      ATR_GND_CTRL = 0;
      VENT_PACE_CTRL = 0;
      ATR_PACE_CTRL = 1;
    state Discharging2
      PACE_CHARGE_CTRL = 0;
      PACE_GND_CTRL = 1;
      VENT_GND_CTRL = 0;
      ATR_GND_CTRL = 0;
      ATR_PACE_CTRL = 0;
      VENT_PACE_CTRL = 1;
    DOO.Charging2 -> (junction 360) [order 2] : [button == true]
    (junction 360) -> DOO.Discharging : [after(lower_interval_rate-ARP,msec)]
    (default) -> DOO.Discharging
    DOO.Discharging2 -> DOO.Charging3 : [after(vent_pulse_width,msec)]
    DOO.Discharging -> DOO.Charging2 : [after(atr_pulse_width,msec)]
    DOO.Charging2 -> DOO.Discharging2 [order 1] : [button == false && after(AV_Delay,msec)]
    DOO.Charging3 -> DOO.Discharging : [after((lower_interval_rate-atr_pulse_width)-AV_Delay-vent_pulse_width,msec)]
  VVI -> INIT : [mode ~= 4]
  AAI -> INIT : [mode ~= 3]
  DDD -> INIT : [mode ~= 5]
  INIT -> DDD [order 6] : [mode == 5]
  INIT -> VVI [order 2] : [mode == 4]
  INIT -> AAI [order 4] : [mode == 3]
  (default) -> INIT
  INIT -> VOO [order 1] : [mode == 2]
  INIT -> AOO [order 3] : [mode == 1]
  AOO -> INIT : [mode ~= 1]
  DOO -> INIT : [mode ~= 0]
  VOO -> INIT : [mode ~= 2]
  INIT -> DOO [order 5] : [mode == 0]
  data: mode input; atr_pulse_width input; PACING_REF_PWM output; Z_ATR_CTRL output; Z_VENT_CTRL output; ATR_PACE_CTRL output; VENT_PACE_CTRL output; PACE_GND_CTRL output; ATR_GND_CTRL output; VENT_GND_CTRL output; PACE_CHARGE_CTRL output; LED_STATE_RED output; LED_STATE_GREEN output; LED_STATE_BLUE output; FRONTEND_CTRL output; atr_amp input; vent_pulse_width input; vent_amp input; upper_interval_rate input; ARP input; VRP input; ATR_CMP_DETECT input; VENT_CMP_DETECT input; lower_interval_rate input; AV_Delay input; HIGH local =true; LOW local =false; button input

== stateflow chart code_group35/rate adaptive/DPR to CPR ==
  state Start
    CPR = LRL
    diff = MSR-LRL
    rate_up = diff/reaction_time
    rate_down = diff/recovery_time
  state edgecase
    if (abs(DPR-CPR) < rate_up | abs(DPR-CPR) < rate_down )
    CPR = DPR
    end
  state UP
  state DOWN
  state Start1 [commented out]
    CPR = 60
    diff = 60
    rate_up = 2
    rate_down = 2
  state edgecase1 [commented out]
    led_green = 1
    led_red = 0
    led_blue = 1
  state UP1 [commented out]
  state DOWN1 [commented out]
    CPR = CPR - rate_down
  (default) -> Start
  Start -> Start [order 2] : [DPR == CPR]
  Start -> edgecase [order 1] : [DPR ~= CPR]
  edgecase -> UP [order 1] : [CPR < DPR]{CPR = CPR + rate_up}
  edgecase -> DOWN [order 2] : [CPR > DPR]{CPR = CPR - rate_down}
  UP -> edgecase : [after(1000,msec)]
  DOWN -> edgecase : [after(1000,msec)]
  (default) -> Start1 [commented out]
  Start1 -> edgecase1 [commented out]
  edgecase1 -> UP1 [commented out] : [CPR < DPR]
  edgecase1 -> DOWN1 [commented out] : [CPR > DPR]
  UP1 -> edgecase1 [commented out] : [after(1000,msec)]
  DOWN1 -> edgecase1 [commented out] : [after(1000,msec)]
  data: DPR input uint32; reaction_time input; recovery_time input; diff local; rate_down local; rate_up local; MSR input; LRL input; CPR output uint32

== matlab function code_group35/rate adaptive/Norm ==
  data: u input; y output
function y = fcn(u)
y = sqrt(u(1)^2+u(2)^2+u(3)^2);
